simulink model "sampleModel2431_slicer"  (R2018a)
settings: Solver=FixedStepAuto  StartTime=0.0  StopTime=10.0  RelTol=1e-3
undefined symbols (not defined in the file): DiscIntNeverNeededParam, sigbuilder_block
libraries: simulink x433
(part 4 of 8)

== system sampleModel2431_slicer/cfblk240 ==
  cfblk1 : Inport
  cfblk13 : Inport  Port=2
  cfblk14 : Inport  Port=3
  Action Port : ActionPort  ActionType=else
  cfblk10 : DiscreteTransferFcn
  cfblk11 : UnitDelay  SampleTime=-1
  cfblk12 : If  SampleTime=1
  cfblk18 : Subsystem  TreatAsAtomicUnit=on
  cfblk19 : Subsystem  TreatAsAtomicUnit=on
  cfblk20 : Delay
  cfblk21 : Delay
  cfblk3 : simulink/Continuous/PID Controller (2DOF)  Controller=PID  TimeDomain=Discrete-time  SampleTime=-1  IntegratorMethod=Forward Euler  FilterMethod=Forward Euler  Form=Parallel  UseFilter=on  ControllerParametersSource=internal  P=1  I=1  D=0  N=100  b=1  c=1  InitialConditionSource=internal  InitialConditionForIntegrator=0  InitialConditionForFilter=0  ExternalReset=none  LimitOutput=off  UpperSaturationLimit=inf  LowerSaturationLimit=-inf  LinearizeAsGain=off  AntiWindupMode=none  Kb=1  TrackingMode=off  Kt=1  PParamMin=[]  PParamMax=[]  IParamMin=[]  IParamMax=[]  DParamMin=[]  DParamMax=[]  NParamMin=[]  NParamMax=[]  bParamMin=[]  bParamMax=[]  cParamMin=[]  cParamMax=[]  KbParamMin=[]  KbParamMax=[]  KtParamMin=[]  KtParamMax=[]  POutMin=[]  POutMax=[]  IOutMin=[]  IOutMax=[]  DOutMin=[]  DOutMax=[]  NOutMin=[]  NOutMax=[]  bOutMin=[]  bOutMax=[]  cOutMin=[]  cOutMax=[]  KbOutMin=[]  KbOutMax=[]  KtOutMin=[]  KtOutMax=[]  IntegratorOutMin=[]  IntegratorOutMax=[]  FilterOutMin=[]  FilterOutMax=[]  SumOutMin=[]  SumOutMax=[]  Sum1OutMin=[]  Sum1OutMax=[]  Sum2OutMin=[]  Sum2OutMax=[]  Sum3OutMin=[]  Sum3OutMax=[]  SumI1OutMin=[]  SumI1OutMax=[]  SumI2OutMin=[]  SumI2OutMax=[]  SumI3OutMin=[]  SumI3OutMax=[]  SumDOutMin=[]  SumDOutMax=[]  SaturationOutMin=[]  SaturationOutMax=[]  IntegratorContinuousStateAttributes=''  IntegratorStateMustResolveToSignalObject=off  IntegratorRTWStateStorageClass=Auto  FilterContinuousStateAttributes=''  FilterStateMustResolveToSignalObject=off  FilterRTWStateStorageClass=Auto  DifferentiatorICPrevScaledInput=0  DifferentiatorOutMin=[]  DifferentiatorOutMax=[]  FilterDiffOutCoefMin=[]  FilterDiffOutCoefMax=[]  SumDenOutMin=[]  SumDenOutMax=[]  SumNumOutMin=[]  SumNumOutMax=[]  ReciprocalOutMin=[]  ReciprocalOutMax=[]  DivideOutMin=[]  DivideOutMax=[]  TunerSelectOption=Transfer Function Based (PID Tuner App)
  cfblk4 : simulink/Discrete/Transfer Fcn First Order  PoleZ=0.95  ICPrevOutput=0.0  DoSatur=off
      settings: SourceProductName=Simulink
  cfblk5 : DiscreteFilter
  cfblk6 : Delay  ShowEnablePort=on
      settings: InputPortMap=u0,e6
  cfblk7 : simulink/Continuous/PID Controller (2DOF)  Controller=PID  TimeDomain=Discrete-time  SampleTime=-1  IntegratorMethod=Forward Euler  FilterMethod=Forward Euler  Form=Parallel  UseFilter=on  ControllerParametersSource=internal  P=1  I=1  D=0  N=100  b=1  c=1  InitialConditionSource=internal  InitialConditionForIntegrator=0  InitialConditionForFilter=0  ExternalReset=none  LimitOutput=off  UpperSaturationLimit=inf  LowerSaturationLimit=-inf  LinearizeAsGain=off  AntiWindupMode=none  Kb=1  TrackingMode=off  Kt=1  PParamMin=[]  PParamMax=[]  IParamMin=[]  IParamMax=[]  DParamMin=[]  DParamMax=[]  NParamMin=[]  NParamMax=[]  bParamMin=[]  bParamMax=[]  cParamMin=[]  cParamMax=[]  KbParamMin=[]  KbParamMax=[]  KtParamMin=[]  KtParamMax=[]  POutMin=[]  POutMax=[]  IOutMin=[]  IOutMax=[]  DOutMin=[]  DOutMax=[]  NOutMin=[]  NOutMax=[]  bOutMin=[]  bOutMax=[]  cOutMin=[]  cOutMax=[]  KbOutMin=[]  KbOutMax=[]  KtOutMin=[]  KtOutMax=[]  IntegratorOutMin=[]  IntegratorOutMax=[]  FilterOutMin=[]  FilterOutMax=[]  SumOutMin=[]  SumOutMax=[]  Sum1OutMin=[]  Sum1OutMax=[]  Sum2OutMin=[]  Sum2OutMax=[]  Sum3OutMin=[]  Sum3OutMax=[]  SumI1OutMin=[]  SumI1OutMax=[]  SumI2OutMin=[]  SumI2OutMax=[]  SumI3OutMin=[]  SumI3OutMax=[]  SumDOutMin=[]  SumDOutMax=[]  SaturationOutMin=[]  SaturationOutMax=[]  IntegratorContinuousStateAttributes=''  IntegratorStateMustResolveToSignalObject=off  IntegratorRTWStateStorageClass=Auto  FilterContinuousStateAttributes=''  FilterStateMustResolveToSignalObject=off  FilterRTWStateStorageClass=Auto  DifferentiatorICPrevScaledInput=0  DifferentiatorOutMin=[]  DifferentiatorOutMax=[]  FilterDiffOutCoefMin=[]  FilterDiffOutCoefMax=[]  SumDenOutMin=[]  SumDenOutMax=[]  SumNumOutMin=[]  SumNumOutMax=[]  ReciprocalOutMin=[]  ReciprocalOutMax=[]  DivideOutMin=[]  DivideOutMax=[]  TunerSelectOption=Transfer Function Based (PID Tuner App)
  cfblk8 : DiscreteStateSpace  SampleTime=-1
  cfblk9 : DiscreteTransferFcn
  cfblk2 : Outport
  cfblk15 : Outport  Port=2
  cfblk16 : Outport  Port=3
  cfblk17 : Outport  Port=4
  wires:
  cfblk18/1(cfblk2) -> cfblk15/1
  cfblk7/1 -> cfblk11/1
  cfblk4/1 -> cfblk9/1
  cfblk6/1 -> cfblk10/1
  cfblk5/1 -> cfblk17/1, cfblk2/1
  cfblk14/1 -> cfblk19/1(cfblk1)
  cfblk9/1 -> cfblk16/1
  cfblk11/1 -> cfblk5/1
  cfblk3/1 -> cfblk4/1
  cfblk8/1 -> cfblk6/1
  cfblk18/3(cfblk17) -> cfblk8/1
  cfblk13/1 -> cfblk18/1(cfblk1), cfblk3/2
  cfblk19/1(cfblk2) -> cfblk7/1
  cfblk19/2(cfblk7) -> cfblk7/2, cfblk18/2(cfblk15)
  cfblk1/1 -> cfblk3/1
  cfblk12/1 -> cfblk18/Action
  cfblk12/2 -> cfblk19/Action
  cfblk10/1 -> cfblk20/1
  cfblk20/1 -> cfblk6/2
  cfblk18/2(cfblk16) -> cfblk21/1
  cfblk21/1 -> cfblk12/1

== system sampleModel2431_slicer/cfblk241 ==
  cfblk1 : Inport
  cfblk9 : Inport  Port=2
  Action Port : ActionPort  ActionType=then
  cfblk11 : Delay
  cfblk3 : Delay  ShowEnablePort=on
      settings: InputPortMap=u0,e6
  cfblk4 : Delay  DelayLengthSource=Input port
      settings: InputPortMap=u0,p1
  cfblk5 : Delay  ShowEnablePort=on
      settings: InputPortMap=u0,e6
  cfblk6 : DiscreteFir
  cfblk7 : simulink/Discrete/Transfer Fcn First Order  PoleZ=0.95  ICPrevOutput=0.0  DoSatur=off
      settings: SourceProductName=Simulink
  cfblk8 : simulink/Discrete/Difference  ICPrevInput=0.0  OutMin=[]  OutMax=[]  OutDataTypeStr=Inherit: Inherit via back propagation  OutDataType=fixdt(1, 16)  OutScaling=2^-10  DoSatur=off
  cfblk2 : Outport
  cfblk10 : Outport  Port=2
  wires:
  cfblk5/1 -> cfblk6/1, cfblk8/1, cfblk10/1
  cfblk3/1 -> cfblk4/1
  cfblk9/1 -> cfblk7/1, cfblk3/2
  cfblk8/1 -> cfblk3/1
  cfblk1/1 -> cfblk4/2
  cfblk4/1 -> cfblk2/1
  cfblk7/1 -> cfblk5/2
  cfblk6/1 -> cfblk11/1
  cfblk11/1 -> cfblk5/1

== system sampleModel2431_slicer/cfblk242 ==
  cfblk1 : Inport
  Action Port : ActionPort  ActionType=else
  cfblk3 : simulink/Continuous/PID Controller  Controller=PID  TimeDomain=Discrete-time  SampleTime=-1  IntegratorMethod=Forward Euler  FilterMethod=Forward Euler  Form=Parallel  UseFilter=on  ControllerParametersSource=internal  P=1  I=1  D=0  N=100  InitialConditionSource=internal  InitialConditionForIntegrator=0  InitialConditionForFilter=0  ExternalReset=none  LimitOutput=off  UpperSaturationLimit=inf  LowerSaturationLimit=-inf  LinearizeAsGain=off  AntiWindupMode=none  Kb=1  TrackingMode=off  Kt=1  PParamMin=[]  PParamMax=[]  IParamMin=[]  IParamMax=[]  DParamMin=[]  DParamMax=[]  NParamMin=[]  NParamMax=[]  KbParamMin=[]  KbParamMax=[]  KtParamMin=[]  KtParamMax=[]  POutMin=[]  POutMax=[]  IOutMin=[]  IOutMax=[]  DOutMin=[]  DOutMax=[]  NOutMin=[]  NOutMax=[]  KbOutMin=[]  KbOutMax=[]  KtOutMin=[]  KtOutMax=[]  IntegratorOutMin=[]  IntegratorOutMax=[]  FilterOutMin=[]  FilterOutMax=[]  SumOutMin=[]  SumOutMax=[]  SumI1OutMin=[]  SumI1OutMax=[]  SumI2OutMin=[]  SumI2OutMax=[]  SumI3OutMin=[]  SumI3OutMax=[]  SumDOutMin=[]  SumDOutMax=[]  SaturationOutMin=[]  SaturationOutMax=[]  IntegratorContinuousStateAttributes=''  IntegratorStateMustResolveToSignalObject=off  IntegratorRTWStateStorageClass=Auto  FilterContinuousStateAttributes=''  FilterStateMustResolveToSignalObject=off  FilterRTWStateStorageClass=Auto  DifferentiatorICPrevScaledInput=0  DifferentiatorOutMin=[]  DifferentiatorOutMax=[]  FilterDiffOutCoefMin=[]  FilterDiffOutCoefMax=[]  SumDenOutMin=[]  SumDenOutMax=[]  SumNumOutMin=[]  SumNumOutMax=[]  ReciprocalOutMin=[]  ReciprocalOutMax=[]  DivideOutMin=[]  DivideOutMax=[]  TunerSelectOption=Transfer Function Based (PID Tuner App)
  cfblk4 : simulink/Discrete/Difference  ICPrevInput=0.0  OutMin=[]  OutMax=[]  OutDataTypeStr=Inherit: Inherit via back propagation  OutDataType=fixdt(1, 16)  OutScaling=2^-10  DoSatur=off
  cfblk5 : DiscreteStateSpace  SampleTime=-1
  cfblk6 : UnitDelay  SampleTime=-1
  cfblk7 : simulink/Discrete/Transfer Fcn Real Zero  ZeroZ=0.75  ICPrevInput=0.0  DoSatur=off
      settings: SourceProductName=Simulink  SourceProductBaseCode=SL
  cfblk8 : Delay
  cfblk9 : Delay
  cfblk2 : Outport
  cfblk10 : Outport  Port=2
  wires:
  cfblk3/1 -> cfblk2/1
  cfblk6/1 -> cfblk7/1
  cfblk4/1 -> cfblk8/1
  cfblk7/1 -> cfblk9/1
  cfblk5/1 -> cfblk4/1
  cfblk1/1 -> cfblk6/1
  cfblk8/1 -> cfblk10/1, cfblk3/1
  cfblk9/1 -> cfblk5/1

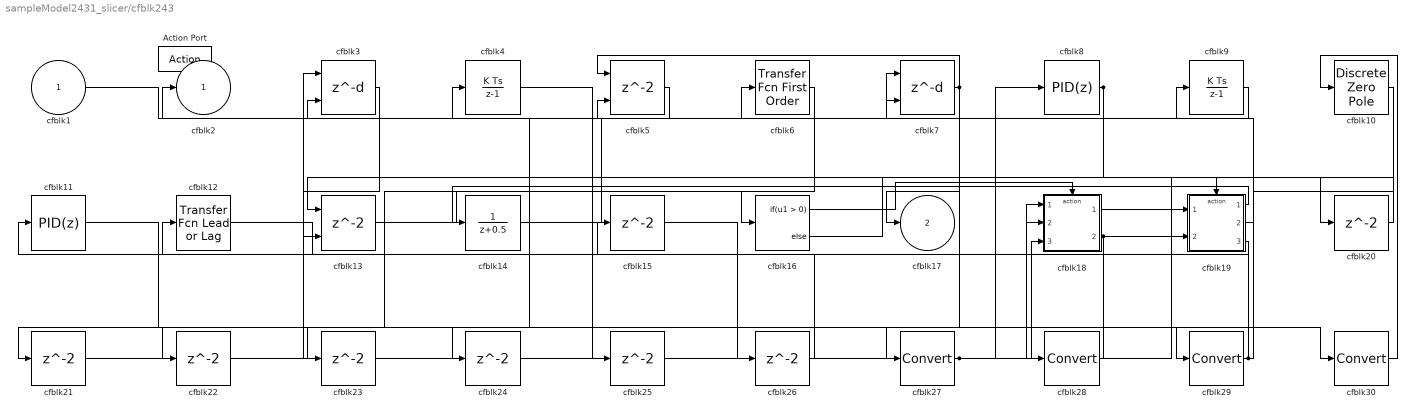
== system sampleModel2431_slicer/cfblk243 ==
  cfblk1 : Inport
  Action Port : ActionPort  ActionType=then
  cfblk10 : DiscreteZeroPole  Poles=[0 0.5]  Gain=1  SampleTime=-1
  cfblk11 : simulink/Continuous/PID Controller  Controller=PID  TimeDomain=Discrete-time  SampleTime=-1  IntegratorMethod=Forward Euler  FilterMethod=Forward Euler  Form=Parallel  UseFilter=on  ControllerParametersSource=internal  P=1  I=1  D=0  N=100  InitialConditionSource=internal  InitialConditionForIntegrator=0  InitialConditionForFilter=0  ExternalReset=none  LimitOutput=off  UpperSaturationLimit=inf  LowerSaturationLimit=-inf  LinearizeAsGain=off  AntiWindupMode=none  Kb=1  TrackingMode=off  Kt=1  PParamMin=[]  PParamMax=[]  IParamMin=[]  IParamMax=[]  DParamMin=[]  DParamMax=[]  NParamMin=[]  NParamMax=[]  KbParamMin=[]  KbParamMax=[]  KtParamMin=[]  KtParamMax=[]  POutMin=[]  POutMax=[]  IOutMin=[]  IOutMax=[]  DOutMin=[]  DOutMax=[]  NOutMin=[]  NOutMax=[]  KbOutMin=[]  KbOutMax=[]  KtOutMin=[]  KtOutMax=[]  IntegratorOutMin=[]  IntegratorOutMax=[]  FilterOutMin=[]  FilterOutMax=[]  SumOutMin=[]  SumOutMax=[]  SumI1OutMin=[]  SumI1OutMax=[]  SumI2OutMin=[]  SumI2OutMax=[]  SumI3OutMin=[]  SumI3OutMax=[]  SumDOutMin=[]  SumDOutMax=[]  SaturationOutMin=[]  SaturationOutMax=[]  IntegratorContinuousStateAttributes=''  IntegratorStateMustResolveToSignalObject=off  IntegratorRTWStateStorageClass=Auto  FilterContinuousStateAttributes=''  FilterStateMustResolveToSignalObject=off  FilterRTWStateStorageClass=Auto  DifferentiatorICPrevScaledInput=0  DifferentiatorOutMin=[]  DifferentiatorOutMax=[]  FilterDiffOutCoefMin=[]  FilterDiffOutCoefMax=[]  SumDenOutMin=[]  SumDenOutMax=[]  SumNumOutMin=[]  SumNumOutMax=[]  ReciprocalOutMin=[]  ReciprocalOutMax=[]  DivideOutMin=[]  DivideOutMax=[]  TunerSelectOption=Transfer Function Based (PID Tuner App)
  cfblk12 : simulink/Discrete/Transfer Fcn Lead or Lag  PoleZ=0.95  ZeroZ=0.75  ICPrevOutput=0.0  ICPrevInput=0.0  DoSatur=off
      settings: SourceProductName=Simulink  SourceProductBaseCode=SL
  cfblk13 : Delay  ShowEnablePort=on
      settings: InputPortMap=u0,e6
  cfblk14 : DiscreteTransferFcn
  cfblk{15,20..26} (8 alike) : Delay
  cfblk16 : If  SampleTime=1
  cfblk18 : Subsystem  TreatAsAtomicUnit=on
  cfblk19 : Subsystem  TreatAsAtomicUnit=on
  cfblk{27..30} (4 alike) : DataTypeConversion
  cfblk3 : Delay  DelayLengthSource=Input port
      settings: InputPortMap=u0,p1
  cfblk4 : DiscreteIntegrator  SampleTime=-1  ICPrevOutput=DiscIntNeverNeededParam  ICPrevScaledInput=DiscIntNeverNeededParam
  cfblk5 : Delay  ShowEnablePort=on
      settings: InputPortMap=u0,e6
  cfblk6 : simulink/Discrete/Transfer Fcn First Order  PoleZ=0.95  ICPrevOutput=0.0  DoSatur=off
      settings: SourceProductName=Simulink
  cfblk7 : Delay  DelayLengthSource=Input port
      settings: InputPortMap=u0,p1
  cfblk8 : simulink/Continuous/PID Controller  Controller=PID  TimeDomain=Discrete-time  SampleTime=-1  IntegratorMethod=Forward Euler  FilterMethod=Forward Euler  Form=Parallel  UseFilter=on  ControllerParametersSource=internal  P=1  I=1  D=0  N=100  InitialConditionSource=internal  InitialConditionForIntegrator=0  InitialConditionForFilter=0  ExternalReset=none  LimitOutput=off  UpperSaturationLimit=inf  LowerSaturationLimit=-inf  LinearizeAsGain=off  AntiWindupMode=none  Kb=1  TrackingMode=off  Kt=1  PParamMin=[]  PParamMax=[]  IParamMin=[]  IParamMax=[]  DParamMin=[]  DParamMax=[]  NParamMin=[]  NParamMax=[]  KbParamMin=[]  KbParamMax=[]  KtParamMin=[]  KtParamMax=[]  POutMin=[]  POutMax=[]  IOutMin=[]  IOutMax=[]  DOutMin=[]  DOutMax=[]  NOutMin=[]  NOutMax=[]  KbOutMin=[]  KbOutMax=[]  KtOutMin=[]  KtOutMax=[]  IntegratorOutMin=[]  IntegratorOutMax=[]  FilterOutMin=[]  FilterOutMax=[]  SumOutMin=[]  SumOutMax=[]  SumI1OutMin=[]  SumI1OutMax=[]  SumI2OutMin=[]  SumI2OutMax=[]  SumI3OutMin=[]  SumI3OutMax=[]  SumDOutMin=[]  SumDOutMax=[]  SaturationOutMin=[]  SaturationOutMax=[]  IntegratorContinuousStateAttributes=''  IntegratorStateMustResolveToSignalObject=off  IntegratorRTWStateStorageClass=Auto  FilterContinuousStateAttributes=''  FilterStateMustResolveToSignalObject=off  FilterRTWStateStorageClass=Auto  DifferentiatorICPrevScaledInput=0  DifferentiatorOutMin=[]  DifferentiatorOutMax=[]  FilterDiffOutCoefMin=[]  FilterDiffOutCoefMax=[]  SumDenOutMin=[]  SumDenOutMax=[]  SumNumOutMin=[]  SumNumOutMax=[]  ReciprocalOutMin=[]  ReciprocalOutMax=[]  DivideOutMin=[]  DivideOutMax=[]  TunerSelectOption=Transfer Function Based (PID Tuner App)
  cfblk9 : DiscreteIntegrator  SampleTime=-1  ICPrevOutput=DiscIntNeverNeededParam  ICPrevScaledInput=DiscIntNeverNeededParam
  cfblk2 : Outport
  cfblk17 : Outport  Port=2
  wires:
  cfblk14/1 -> cfblk7/1
  cfblk12/1 -> cfblk15/1
  cfblk9/1 -> cfblk7/2
  cfblk7/1 -> cfblk5/1, cfblk17/1, cfblk22/1
  cfblk5/1 -> cfblk2/1
  cfblk18/2(cfblk16) -> cfblk19/2(cfblk11), cfblk21/1
  cfblk10/1 -> cfblk29/1
  cfblk11/1 -> cfblk27/1
  cfblk13/1 -> cfblk16/1
  cfblk8/1 -> cfblk5/2, cfblk24/1
  cfblk1/1 -> cfblk3/2
  cfblk3/1 -> cfblk13/2
  cfblk19/1(cfblk2) -> cfblk14/1
  cfblk19/2(cfblk12) -> cfblk6/1
  cfblk16/1 -> cfblk18/Action
  cfblk16/2 -> cfblk19/Action
  cfblk18/1(cfblk2) -> cfblk20/1
  cfblk20/1 -> cfblk13/1
  cfblk21/1 -> cfblk3/1
  cfblk22/1 -> cfblk18/3(cfblk15)
  cfblk6/1 -> cfblk23/1
  cfblk23/1 -> cfblk18/1(cfblk1)
  cfblk24/1 -> cfblk18/2(cfblk14)
  cfblk4/1 -> cfblk25/1
  cfblk25/1 -> cfblk19/1(cfblk1)
  cfblk15/1 -> cfblk26/1
  cfblk26/1 -> cfblk12/1
  cfblk27/1 -> cfblk8/1, cfblk30/1
  cfblk19/3(cfblk13) -> cfblk28/1
  cfblk28/1 -> cfblk11/1
  cfblk29/1 -> cfblk4/1, cfblk9/1
  cfblk30/1 -> cfblk10/1

== system sampleModel2431_slicer/cfblk244 ==
  cfblk1 : Inport
  Action Port : ActionPort  ActionType=else
  cfblk10 : Delay
  cfblk11 : Delay
  cfblk12 : Delay
  cfblk3 : UnitDelay  SampleTime=-1
  cfblk4 : simulink/Discrete/Transfer Fcn Real Zero  ZeroZ=0.75  ICPrevInput=0.0  DoSatur=off
      settings: SourceProductName=Simulink  SourceProductBaseCode=SL
  cfblk5 : simulink/Discrete/Transfer Fcn Lead or Lag  PoleZ=0.95  ZeroZ=0.75  ICPrevOutput=0.0  ICPrevInput=0.0  DoSatur=off
      settings: SourceProductName=Simulink  SourceProductBaseCode=SL
  cfblk6 : DiscreteFir
  cfblk7 : If  SampleTime=1
  cfblk8 : Subsystem  TreatAsAtomicUnit=on
  cfblk9 : Subsystem  TreatAsAtomicUnit=on
  cfblk2 : Outport
  wires:
  cfblk1/1 -> cfblk5/1
  cfblk4/1 -> cfblk3/1, cfblk11/1
  cfblk5/1 -> cfblk2/1, cfblk6/1
  cfblk6/1 -> cfblk8/2(cfblk13)
  cfblk8/1(cfblk2) -> cfblk4/1
  cfblk8/2(cfblk15) -> cfblk9/1(cfblk1)
  cfblk8/3(cfblk16) -> cfblk9/2(cfblk10)
  cfblk7/1 -> cfblk8/Action
  cfblk7/2 -> cfblk9/Action
  cfblk3/1 -> cfblk10/1
  cfblk10/1 -> cfblk8/1(cfblk1)
  cfblk11/1 -> cfblk8/3(cfblk14)
  cfblk9/1(cfblk2) -> cfblk12/1
  cfblk12/1 -> cfblk7/1

== system sampleModel2431_slicer/cfblk245 ==
  cfblk1 : Inport
  cfblk12 : Inport  Port=2
  cfblk13 : Inport  Port=3
  Action Port : ActionPort  ActionType=then
  cfblk10 : If  SampleTime=1
  cfblk11 : If  SampleTime=1
  cfblk14 : Subsystem  TreatAsAtomicUnit=on
  cfblk15 : Subsystem  TreatAsAtomicUnit=on
  cfblk16 : Subsystem  TreatAsAtomicUnit=on
  cfblk17 : Subsystem  TreatAsAtomicUnit=on
  cfblk{18..21} (4 alike) : Delay
  cfblk3 : DiscreteIntegrator  SampleTime=-1  ICPrevOutput=DiscIntNeverNeededParam  ICPrevScaledInput=DiscIntNeverNeededParam
  cfblk4 : simulink/Discrete/Transfer Fcn First Order  PoleZ=0.95  ICPrevOutput=0.0  DoSatur=off
      settings: SourceProductName=Simulink
  cfblk5 : simulink/Discrete/Difference  ICPrevInput=0.0  OutMin=[]  OutMax=[]  OutDataTypeStr=Inherit: Inherit via back propagation  OutDataType=fixdt(1, 16)  OutScaling=2^-10  DoSatur=off
  cfblk6 : DiscreteStateSpace  SampleTime=-1
  cfblk7 : simulink/Discrete/Tapped Delay  vinit=0.0  samptime=-1  NumDelays=1  DelayOrder=Oldest  includeCurrent=off
  cfblk8 : Delay  ShowEnablePort=on
      settings: InputPortMap=u0,e6
  cfblk9 : Delay  ShowEnablePort=on
      settings: InputPortMap=u0,e6
  cfblk2 : Outport
  wires:
  cfblk9/1 -> cfblk6/1
  cfblk7/1 -> cfblk15/1(cfblk1), cfblk8/2, cfblk15/4(cfblk11), cfblk20/1
  cfblk1/1 -> cfblk16/1(cfblk1), cfblk17/3(cfblk16)
  cfblk16/1(cfblk2) -> cfblk10/1
  cfblk12/1 -> cfblk16/2(cfblk8)
  cfblk15/1(cfblk2) -> cfblk5/1
  cfblk3/1 -> cfblk8/1
  cfblk8/1 -> cfblk9/1
  cfblk15/2(cfblk12) -> cfblk3/1
  cfblk4/1 -> cfblk14/1(cfblk1), cfblk7/1
  cfblk13/1 -> cfblk9/2
  cfblk16/2(cfblk9) -> cfblk4/1, cfblk14/2(cfblk11), cfblk21/1
  cfblk14/1(cfblk2) -> cfblk15/3(cfblk10)
  cfblk17/1(cfblk2) -> cfblk2/1
  cfblk10/1 -> cfblk14/Action
  cfblk10/2 -> cfblk15/Action
  cfblk11/1 -> cfblk16/Action
  cfblk11/2 -> cfblk17/Action
  cfblk5/1 -> cfblk18/1
  cfblk18/1 -> cfblk17/1(cfblk1)
  cfblk6/1 -> cfblk19/1
  cfblk19/1 -> cfblk15/2(cfblk9)
  cfblk20/1 -> cfblk17/2(cfblk15)
  cfblk21/1 -> cfblk11/1

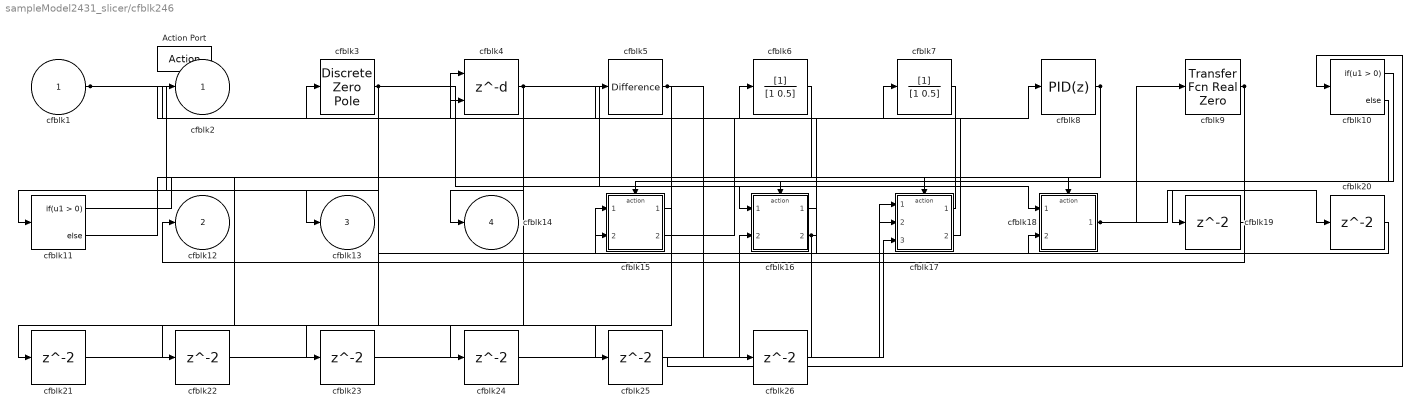
== system sampleModel2431_slicer/cfblk246 ==
  cfblk1 : Inport
  Action Port : ActionPort  ActionType=else
  cfblk10 : If  SampleTime=1
  cfblk11 : If  SampleTime=1
  cfblk15 : Subsystem  TreatAsAtomicUnit=on
  cfblk16 : Subsystem  TreatAsAtomicUnit=on
  cfblk17 : Subsystem  TreatAsAtomicUnit=on
  cfblk18 : Subsystem  TreatAsAtomicUnit=on
  cfblk{19..26} (8 alike) : Delay
  cfblk3 : DiscreteZeroPole  Poles=[0 0.5]  Gain=1  SampleTime=-1
  cfblk4 : Delay  DelayLengthSource=Input port
      settings: InputPortMap=u0,p1
  cfblk5 : simulink/Discrete/Difference  ICPrevInput=0.0  OutMin=[]  OutMax=[]  OutDataTypeStr=Inherit: Inherit via back propagation  OutDataType=fixdt(1, 16)  OutScaling=2^-10  DoSatur=off
  cfblk6 : DiscreteFilter
  cfblk7 : DiscreteFilter
  cfblk8 : simulink/Continuous/PID Controller  Controller=PID  TimeDomain=Discrete-time  SampleTime=-1  IntegratorMethod=Forward Euler  FilterMethod=Forward Euler  Form=Parallel  UseFilter=on  ControllerParametersSource=internal  P=1  I=1  D=0  N=100  InitialConditionSource=internal  InitialConditionForIntegrator=0  InitialConditionForFilter=0  ExternalReset=none  LimitOutput=off  UpperSaturationLimit=inf  LowerSaturationLimit=-inf  LinearizeAsGain=off  AntiWindupMode=none  Kb=1  TrackingMode=off  Kt=1  PParamMin=[]  PParamMax=[]  IParamMin=[]  IParamMax=[]  DParamMin=[]  DParamMax=[]  NParamMin=[]  NParamMax=[]  KbParamMin=[]  KbParamMax=[]  KtParamMin=[]  KtParamMax=[]  POutMin=[]  POutMax=[]  IOutMin=[]  IOutMax=[]  DOutMin=[]  DOutMax=[]  NOutMin=[]  NOutMax=[]  KbOutMin=[]  KbOutMax=[]  KtOutMin=[]  KtOutMax=[]  IntegratorOutMin=[]  IntegratorOutMax=[]  FilterOutMin=[]  FilterOutMax=[]  SumOutMin=[]  SumOutMax=[]  SumI1OutMin=[]  SumI1OutMax=[]  SumI2OutMin=[]  SumI2OutMax=[]  SumI3OutMin=[]  SumI3OutMax=[]  SumDOutMin=[]  SumDOutMax=[]  SaturationOutMin=[]  SaturationOutMax=[]  IntegratorContinuousStateAttributes=''  IntegratorStateMustResolveToSignalObject=off  IntegratorRTWStateStorageClass=Auto  FilterContinuousStateAttributes=''  FilterStateMustResolveToSignalObject=off  FilterRTWStateStorageClass=Auto  DifferentiatorICPrevScaledInput=0  DifferentiatorOutMin=[]  DifferentiatorOutMax=[]  FilterDiffOutCoefMin=[]  FilterDiffOutCoefMax=[]  SumDenOutMin=[]  SumDenOutMax=[]  SumNumOutMin=[]  SumNumOutMax=[]  ReciprocalOutMin=[]  ReciprocalOutMax=[]  DivideOutMin=[]  DivideOutMax=[]  TunerSelectOption=Transfer Function Based (PID Tuner App)
  cfblk9 : simulink/Discrete/Transfer Fcn Real Zero  ZeroZ=0.75  ICPrevInput=0.0  DoSatur=off
      settings: SourceProductName=Simulink  SourceProductBaseCode=SL
  cfblk2 : Outport
  cfblk12 : Outport  Port=2
  cfblk13 : Outport  Port=3
  cfblk14 : Outport  Port=4
  wires:
  cfblk1/1 -> cfblk13/1, cfblk4/1
  cfblk4/1 -> cfblk16/1(cfblk1), cfblk14/1
  cfblk16/1(cfblk2) -> cfblk3/1
  cfblk8/1 -> cfblk23/1, cfblk24/1
  cfblk15/2(cfblk12) -> cfblk8/1
  cfblk5/1 -> cfblk25/1, cfblk26/1
  cfblk16/2(cfblk17) -> cfblk5/1, cfblk15/1(cfblk1)
  cfblk7/1 -> cfblk2/1
  cfblk18/1(cfblk2) -> cfblk9/1, cfblk20/1
  cfblk9/1 -> cfblk12/1, cfblk19/1
  cfblk17/1(cfblk2) -> cfblk6/1
  cfblk3/1 -> cfblk18/1(cfblk1), cfblk11/1
  cfblk17/2(cfblk9) -> cfblk7/1
  cfblk10/1 -> cfblk15/Action
  cfblk10/2 -> cfblk16/Action
  cfblk11/1 -> cfblk17/Action
  cfblk11/2 -> cfblk18/Action
  cfblk19/1 -> cfblk18/2(cfblk10)
  cfblk20/1 -> cfblk15/2(cfblk11)
  cfblk15/1(cfblk2) -> cfblk21/1
  cfblk21/1 -> cfblk17/1(cfblk1)
  cfblk6/1 -> cfblk22/1
  cfblk22/1 -> cfblk17/2(cfblk7)
  cfblk23/1 -> cfblk17/3(cfblk8)
  cfblk24/1 -> cfblk16/2(cfblk16)
  cfblk25/1 -> cfblk10/1
  cfblk26/1 -> cfblk4/2

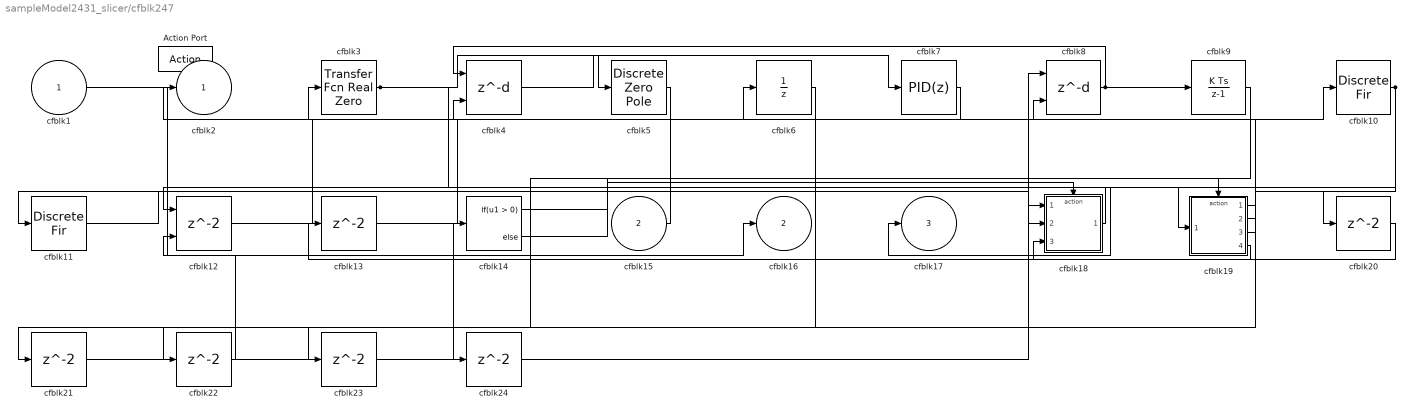
== system sampleModel2431_slicer/cfblk247 ==
  cfblk1 : Inport
  cfblk15 : Inport  Port=2
  Action Port : ActionPort  ActionType=then
  cfblk10 : DiscreteFir
  cfblk11 : DiscreteFir
  cfblk12 : Delay  ShowEnablePort=on
      settings: InputPortMap=u0,e6
  cfblk{13,20..24} (6 alike) : Delay
  cfblk14 : If  SampleTime=1
  cfblk18 : Subsystem  TreatAsAtomicUnit=on
  cfblk19 : Subsystem  TreatAsAtomicUnit=on
  cfblk3 : simulink/Discrete/Transfer Fcn Real Zero  ZeroZ=0.75  ICPrevInput=0.0  DoSatur=off
      settings: SourceProductName=Simulink  SourceProductBaseCode=SL
  cfblk4 : Delay  DelayLengthSource=Input port
      settings: InputPortMap=u0,p1
  cfblk5 : DiscreteZeroPole  Poles=[0 0.5]  Gain=1  SampleTime=-1
  cfblk6 : UnitDelay  SampleTime=-1
  cfblk7 : simulink/Continuous/PID Controller  Controller=PID  TimeDomain=Discrete-time  SampleTime=-1  IntegratorMethod=Forward Euler  FilterMethod=Forward Euler  Form=Parallel  UseFilter=on  ControllerParametersSource=internal  P=1  I=1  D=0  N=100  InitialConditionSource=internal  InitialConditionForIntegrator=0  InitialConditionForFilter=0  ExternalReset=none  LimitOutput=off  UpperSaturationLimit=inf  LowerSaturationLimit=-inf  LinearizeAsGain=off  AntiWindupMode=none  Kb=1  TrackingMode=off  Kt=1  PParamMin=[]  PParamMax=[]  IParamMin=[]  IParamMax=[]  DParamMin=[]  DParamMax=[]  NParamMin=[]  NParamMax=[]  KbParamMin=[]  KbParamMax=[]  KtParamMin=[]  KtParamMax=[]  POutMin=[]  POutMax=[]  IOutMin=[]  IOutMax=[]  DOutMin=[]  DOutMax=[]  NOutMin=[]  NOutMax=[]  KbOutMin=[]  KbOutMax=[]  KtOutMin=[]  KtOutMax=[]  IntegratorOutMin=[]  IntegratorOutMax=[]  FilterOutMin=[]  FilterOutMax=[]  SumOutMin=[]  SumOutMax=[]  SumI1OutMin=[]  SumI1OutMax=[]  SumI2OutMin=[]  SumI2OutMax=[]  SumI3OutMin=[]  SumI3OutMax=[]  SumDOutMin=[]  SumDOutMax=[]  SaturationOutMin=[]  SaturationOutMax=[]  IntegratorContinuousStateAttributes=''  IntegratorStateMustResolveToSignalObject=off  IntegratorRTWStateStorageClass=Auto  FilterContinuousStateAttributes=''  FilterStateMustResolveToSignalObject=off  FilterRTWStateStorageClass=Auto  DifferentiatorICPrevScaledInput=0  DifferentiatorOutMin=[]  DifferentiatorOutMax=[]  FilterDiffOutCoefMin=[]  FilterDiffOutCoefMax=[]  SumDenOutMin=[]  SumDenOutMax=[]  SumNumOutMin=[]  SumNumOutMax=[]  ReciprocalOutMin=[]  ReciprocalOutMax=[]  DivideOutMin=[]  DivideOutMax=[]  TunerSelectOption=Transfer Function Based (PID Tuner App)
  cfblk8 : Delay  DelayLengthSource=Input port
      settings: InputPortMap=u0,p1
  cfblk9 : DiscreteIntegrator  SampleTime=-1  ICPrevOutput=DiscIntNeverNeededParam  ICPrevScaledInput=DiscIntNeverNeededParam
  cfblk2 : Outport
  cfblk16 : Outport  Port=2
  cfblk17 : Outport  Port=3
  wires:
  cfblk12/1 -> cfblk10/1
  cfblk15/1 -> cfblk3/1
  cfblk3/1 -> cfblk5/1, cfblk19/1(cfblk1)
  cfblk1/1 -> cfblk16/1
  cfblk8/1 -> cfblk4/1, cfblk9/1
  cfblk10/1 -> cfblk17/1, cfblk20/1, cfblk21/1
  cfblk18/1(cfblk2) -> cfblk12/1
  cfblk4/1 -> cfblk7/1
  cfblk5/1 -> cfblk11/1
  cfblk11/1 -> cfblk18/2(cfblk11)
  cfblk7/1 -> cfblk2/1
  cfblk19/2(cfblk5) -> cfblk4/2
  cfblk13/1 -> cfblk8/2
  cfblk19/3(cfblk6) -> cfblk6/1
  cfblk19/4(cfblk7) -> cfblk13/1
  cfblk14/1 -> cfblk18/Action
  cfblk14/2 -> cfblk19/Action
  cfblk20/1 -> cfblk18/3(cfblk12)
  cfblk21/1 -> cfblk14/1
  cfblk19/1(cfblk2) -> cfblk22/1
  cfblk22/1 -> cfblk12/2
  cfblk6/1 -> cfblk23/1
  cfblk23/1 -> cfblk18/1(cfblk1)
  cfblk9/1 -> cfblk24/1
  cfblk24/1 -> cfblk8/1

== system sampleModel2431_slicer/cfblk248 ==
  cfblk1 : Inport
  cfblk8 : Inport  Port=2
  Action Port : ActionPort  ActionType=else
  cfblk3 : Delay  ShowEnablePort=on
      settings: InputPortMap=u0,e6
  cfblk4 : Delay  DelayLengthSource=Input port
      settings: InputPortMap=u0,p1
  cfblk5 : Delay
  cfblk6 : DiscreteStateSpace  SampleTime=-1
  cfblk7 : simulink/Discrete/Transfer Fcn Lead or Lag  PoleZ=0.95  ZeroZ=0.75  ICPrevOutput=0.0  ICPrevInput=0.0  DoSatur=off
      settings: SourceProductName=Simulink  SourceProductBaseCode=SL
  cfblk2 : Outport
  cfblk9 : Outport  Port=2
  wires:
  cfblk7/1 -> cfblk4/1, cfblk4/2
  cfblk4/1 -> cfblk9/1
  cfblk8/1 -> cfblk6/1
  cfblk6/1 -> cfblk3/1, cfblk3/2
  cfblk1/1 -> cfblk2/1
  cfblk3/1 -> cfblk5/1
  cfblk5/1 -> cfblk7/1

== system sampleModel2431_slicer/cfblk249 ==
  cfblk1 : Inport
  cfblk12 : Inport  Port=2
  Action Port : ActionPort  ActionType=then
  cfblk10 : DiscreteFilter
  cfblk11 : DiscreteTransferFcn
  cfblk13 : Delay
  cfblk3 : Delay
  cfblk4 : simulink/Discrete/Difference  ICPrevInput=0.0  OutMin=[]  OutMax=[]  OutDataTypeStr=Inherit: Inherit via back propagation  OutDataType=fixdt(1, 16)  OutScaling=2^-10  DoSatur=off
  cfblk5 : simulink/Discrete/Transfer Fcn Lead or Lag  PoleZ=0.95  ZeroZ=0.75  ICPrevOutput=0.0  ICPrevInput=0.0  DoSatur=off
      settings: SourceProductName=Simulink  SourceProductBaseCode=SL
  cfblk6 : DiscreteFir
  cfblk7 : DiscreteIntegrator  SampleTime=-1  ICPrevOutput=DiscIntNeverNeededParam  ICPrevScaledInput=DiscIntNeverNeededParam
  cfblk8 : simulink/Continuous/PID Controller  Controller=PID  TimeDomain=Discrete-time  SampleTime=-1  IntegratorMethod=Forward Euler  FilterMethod=Forward Euler  Form=Parallel  UseFilter=on  ControllerParametersSource=internal  P=1  I=1  D=0  N=100  InitialConditionSource=internal  InitialConditionForIntegrator=0  InitialConditionForFilter=0  ExternalReset=none  LimitOutput=off  UpperSaturationLimit=inf  LowerSaturationLimit=-inf  LinearizeAsGain=off  AntiWindupMode=none  Kb=1  TrackingMode=off  Kt=1  PParamMin=[]  PParamMax=[]  IParamMin=[]  IParamMax=[]  DParamMin=[]  DParamMax=[]  NParamMin=[]  NParamMax=[]  KbParamMin=[]  KbParamMax=[]  KtParamMin=[]  KtParamMax=[]  POutMin=[]  POutMax=[]  IOutMin=[]  IOutMax=[]  DOutMin=[]  DOutMax=[]  NOutMin=[]  NOutMax=[]  KbOutMin=[]  KbOutMax=[]  KtOutMin=[]  KtOutMax=[]  IntegratorOutMin=[]  IntegratorOutMax=[]  FilterOutMin=[]  FilterOutMax=[]  SumOutMin=[]  SumOutMax=[]  SumI1OutMin=[]  SumI1OutMax=[]  SumI2OutMin=[]  SumI2OutMax=[]  SumI3OutMin=[]  SumI3OutMax=[]  SumDOutMin=[]  SumDOutMax=[]  SaturationOutMin=[]  SaturationOutMax=[]  IntegratorContinuousStateAttributes=''  IntegratorStateMustResolveToSignalObject=off  IntegratorRTWStateStorageClass=Auto  FilterContinuousStateAttributes=''  FilterStateMustResolveToSignalObject=off  FilterRTWStateStorageClass=Auto  DifferentiatorICPrevScaledInput=0  DifferentiatorOutMin=[]  DifferentiatorOutMax=[]  FilterDiffOutCoefMin=[]  FilterDiffOutCoefMax=[]  SumDenOutMin=[]  SumDenOutMax=[]  SumNumOutMin=[]  SumNumOutMax=[]  ReciprocalOutMin=[]  ReciprocalOutMax=[]  DivideOutMin=[]  DivideOutMax=[]  TunerSelectOption=Transfer Function Based (PID Tuner App)
  cfblk9 : DiscreteStateSpace  SampleTime=-1
  cfblk2 : Outport
  wires:
  cfblk1/1 -> cfblk7/1
  cfblk10/1 -> cfblk2/1
  cfblk11/1 -> cfblk6/1
  cfblk12/1 -> cfblk11/1
  cfblk7/1 -> cfblk4/1
  cfblk4/1 -> cfblk9/1
  cfblk5/1 -> cfblk8/1
  cfblk3/1 -> cfblk10/1
  cfblk6/1 -> cfblk3/1
  cfblk8/1 -> cfblk13/1
  cfblk13/1 -> cfblk5/1

== system sampleModel2431_slicer/cfblk250 ==
  cfblk1 : Inport
  cfblk12 : Inport  Port=2
  cfblk13 : Inport  Port=3
  cfblk14 : Inport  Port=4
  Action Port : ActionPort  ActionType=else
  cfblk10 : DiscreteTransferFcn
  cfblk11 : If  SampleTime=1
  cfblk16 : Subsystem  TreatAsAtomicUnit=on
  cfblk17 : Subsystem  TreatAsAtomicUnit=on
  cfblk18 : Delay
  cfblk3 : DiscreteIntegrator  SampleTime=-1  ICPrevOutput=DiscIntNeverNeededParam  ICPrevScaledInput=DiscIntNeverNeededParam
  cfblk4 : simulink/Continuous/PID Controller (2DOF)  Controller=PID  TimeDomain=Discrete-time  SampleTime=-1  IntegratorMethod=Forward Euler  FilterMethod=Forward Euler  Form=Parallel  UseFilter=on  ControllerParametersSource=internal  P=1  I=1  D=0  N=100  b=1  c=1  InitialConditionSource=internal  InitialConditionForIntegrator=0  InitialConditionForFilter=0  ExternalReset=none  LimitOutput=off  UpperSaturationLimit=inf  LowerSaturationLimit=-inf  LinearizeAsGain=off  AntiWindupMode=none  Kb=1  TrackingMode=off  Kt=1  PParamMin=[]  PParamMax=[]  IParamMin=[]  IParamMax=[]  DParamMin=[]  DParamMax=[]  NParamMin=[]  NParamMax=[]  bParamMin=[]  bParamMax=[]  cParamMin=[]  cParamMax=[]  KbParamMin=[]  KbParamMax=[]  KtParamMin=[]  KtParamMax=[]  POutMin=[]  POutMax=[]  IOutMin=[]  IOutMax=[]  DOutMin=[]  DOutMax=[]  NOutMin=[]  NOutMax=[]  bOutMin=[]  bOutMax=[]  cOutMin=[]  cOutMax=[]  KbOutMin=[]  KbOutMax=[]  KtOutMin=[]  KtOutMax=[]  IntegratorOutMin=[]  IntegratorOutMax=[]  FilterOutMin=[]  FilterOutMax=[]  SumOutMin=[]  SumOutMax=[]  Sum1OutMin=[]  Sum1OutMax=[]  Sum2OutMin=[]  Sum2OutMax=[]  Sum3OutMin=[]  Sum3OutMax=[]  SumI1OutMin=[]  SumI1OutMax=[]  SumI2OutMin=[]  SumI2OutMax=[]  SumI3OutMin=[]  SumI3OutMax=[]  SumDOutMin=[]  SumDOutMax=[]  SaturationOutMin=[]  SaturationOutMax=[]  IntegratorContinuousStateAttributes=''  IntegratorStateMustResolveToSignalObject=off  IntegratorRTWStateStorageClass=Auto  FilterContinuousStateAttributes=''  FilterStateMustResolveToSignalObject=off  FilterRTWStateStorageClass=Auto  DifferentiatorICPrevScaledInput=0  DifferentiatorOutMin=[]  DifferentiatorOutMax=[]  FilterDiffOutCoefMin=[]  FilterDiffOutCoefMax=[]  SumDenOutMin=[]  SumDenOutMax=[]  SumNumOutMin=[]  SumNumOutMax=[]  ReciprocalOutMin=[]  ReciprocalOutMax=[]  DivideOutMin=[]  DivideOutMax=[]  TunerSelectOption=Transfer Function Based (PID Tuner App)
  cfblk5 : DiscreteIntegrator  SampleTime=-1  ICPrevOutput=DiscIntNeverNeededParam  ICPrevScaledInput=DiscIntNeverNeededParam
  cfblk6 : simulink/Discrete/Transfer Fcn First Order  PoleZ=0.95  ICPrevOutput=0.0  DoSatur=off
      settings: SourceProductName=Simulink
  cfblk7 : simulink/Continuous/PID Controller (2DOF)  Controller=PID  TimeDomain=Discrete-time  SampleTime=-1  IntegratorMethod=Forward Euler  FilterMethod=Forward Euler  Form=Parallel  UseFilter=on  ControllerParametersSource=internal  P=1  I=1  D=0  N=100  b=1  c=1  InitialConditionSource=internal  InitialConditionForIntegrator=0  InitialConditionForFilter=0  ExternalReset=none  LimitOutput=off  UpperSaturationLimit=inf  LowerSaturationLimit=-inf  LinearizeAsGain=off  AntiWindupMode=none  Kb=1  TrackingMode=off  Kt=1  PParamMin=[]  PParamMax=[]  IParamMin=[]  IParamMax=[]  DParamMin=[]  DParamMax=[]  NParamMin=[]  NParamMax=[]  bParamMin=[]  bParamMax=[]  cParamMin=[]  cParamMax=[]  KbParamMin=[]  KbParamMax=[]  KtParamMin=[]  KtParamMax=[]  POutMin=[]  POutMax=[]  IOutMin=[]  IOutMax=[]  DOutMin=[]  DOutMax=[]  NOutMin=[]  NOutMax=[]  bOutMin=[]  bOutMax=[]  cOutMin=[]  cOutMax=[]  KbOutMin=[]  KbOutMax=[]  KtOutMin=[]  KtOutMax=[]  IntegratorOutMin=[]  IntegratorOutMax=[]  FilterOutMin=[]  FilterOutMax=[]  SumOutMin=[]  SumOutMax=[]  Sum1OutMin=[]  Sum1OutMax=[]  Sum2OutMin=[]  Sum2OutMax=[]  Sum3OutMin=[]  Sum3OutMax=[]  SumI1OutMin=[]  SumI1OutMax=[]  SumI2OutMin=[]  SumI2OutMax=[]  SumI3OutMin=[]  SumI3OutMax=[]  SumDOutMin=[]  SumDOutMax=[]  SaturationOutMin=[]  SaturationOutMax=[]  IntegratorContinuousStateAttributes=''  IntegratorStateMustResolveToSignalObject=off  IntegratorRTWStateStorageClass=Auto  FilterContinuousStateAttributes=''  FilterStateMustResolveToSignalObject=off  FilterRTWStateStorageClass=Auto  DifferentiatorICPrevScaledInput=0  DifferentiatorOutMin=[]  DifferentiatorOutMax=[]  FilterDiffOutCoefMin=[]  FilterDiffOutCoefMax=[]  SumDenOutMin=[]  SumDenOutMax=[]  SumNumOutMin=[]  SumNumOutMax=[]  ReciprocalOutMin=[]  ReciprocalOutMax=[]  DivideOutMin=[]  DivideOutMax=[]  TunerSelectOption=Transfer Function Based (PID Tuner App)
  cfblk8 : simulink/Discrete/Transfer Fcn Real Zero  ZeroZ=0.75  ICPrevInput=0.0  DoSatur=off
      settings: SourceProductName=Simulink  SourceProductBaseCode=SL
  cfblk9 : simulink/Discrete/Transfer Fcn Real Zero  ZeroZ=0.75  ICPrevInput=0.0  DoSatur=off
      settings: SourceProductName=Simulink  SourceProductBaseCode=SL
  cfblk2 : Outport
  cfblk15 : Outport  Port=2
  wires:
  cfblk17/1(cfblk2) -> cfblk10/1
  cfblk17/2(cfblk12) -> cfblk9/1
  cfblk13/1 -> cfblk5/1
  cfblk4/1 -> cfblk8/1
  cfblk6/1 -> cfblk3/1
  cfblk1/1 -> cfblk11/1
  cfblk16/1(cfblk2) -> cfblk6/1
  cfblk10/1 -> cfblk15/1
  cfblk5/1 -> cfblk16/1(cfblk1)
  cfblk14/1 -> cfblk4/1
  cfblk12/1 -> cfblk16/2(cfblk11)
  cfblk9/1 -> cfblk2/1
  cfblk3/1 -> cfblk7/1
  cfblk16/2(cfblk12) -> cfblk4/2, cfblk7/2
  cfblk11/1 -> cfblk16/Action
  cfblk11/2 -> cfblk17/Action
  cfblk8/1 -> cfblk18/1
  cfblk18/1 -> cfblk17/1(cfblk1)

== system sampleModel2431_slicer/cfblk251 ==
  cfblk1 : Inport
  cfblk8 : Inport  Port=2
  Action Port : ActionPort  ActionType=then
  cfblk11 : Subsystem  TreatAsAtomicUnit=on
  cfblk12 : Subsystem  TreatAsAtomicUnit=on
  cfblk13 : Delay
  cfblk14 : Delay
  cfblk3 : Delay
  cfblk4 : DiscreteFir
  cfblk5 : simulink/Discrete/Transfer Fcn First Order  PoleZ=0.95  ICPrevOutput=0.0  DoSatur=off
      settings: SourceProductName=Simulink
  cfblk6 : simulink/Continuous/PID Controller (2DOF)  Controller=PID  TimeDomain=Discrete-time  SampleTime=-1  IntegratorMethod=Forward Euler  FilterMethod=Forward Euler  Form=Parallel  UseFilter=on  ControllerParametersSource=internal  P=1  I=1  D=0  N=100  b=1  c=1  InitialConditionSource=internal  InitialConditionForIntegrator=0  InitialConditionForFilter=0  ExternalReset=none  LimitOutput=off  UpperSaturationLimit=inf  LowerSaturationLimit=-inf  LinearizeAsGain=off  AntiWindupMode=none  Kb=1  TrackingMode=off  Kt=1  PParamMin=[]  PParamMax=[]  IParamMin=[]  IParamMax=[]  DParamMin=[]  DParamMax=[]  NParamMin=[]  NParamMax=[]  bParamMin=[]  bParamMax=[]  cParamMin=[]  cParamMax=[]  KbParamMin=[]  KbParamMax=[]  KtParamMin=[]  KtParamMax=[]  POutMin=[]  POutMax=[]  IOutMin=[]  IOutMax=[]  DOutMin=[]  DOutMax=[]  NOutMin=[]  NOutMax=[]  bOutMin=[]  bOutMax=[]  cOutMin=[]  cOutMax=[]  KbOutMin=[]  KbOutMax=[]  KtOutMin=[]  KtOutMax=[]  IntegratorOutMin=[]  IntegratorOutMax=[]  FilterOutMin=[]  FilterOutMax=[]  SumOutMin=[]  SumOutMax=[]  Sum1OutMin=[]  Sum1OutMax=[]  Sum2OutMin=[]  Sum2OutMax=[]  Sum3OutMin=[]  Sum3OutMax=[]  SumI1OutMin=[]  SumI1OutMax=[]  SumI2OutMin=[]  SumI2OutMax=[]  SumI3OutMin=[]  SumI3OutMax=[]  SumDOutMin=[]  SumDOutMax=[]  SaturationOutMin=[]  SaturationOutMax=[]  IntegratorContinuousStateAttributes=''  IntegratorStateMustResolveToSignalObject=off  IntegratorRTWStateStorageClass=Auto  FilterContinuousStateAttributes=''  FilterStateMustResolveToSignalObject=off  FilterRTWStateStorageClass=Auto  DifferentiatorICPrevScaledInput=0  DifferentiatorOutMin=[]  DifferentiatorOutMax=[]  FilterDiffOutCoefMin=[]  FilterDiffOutCoefMax=[]  SumDenOutMin=[]  SumDenOutMax=[]  SumNumOutMin=[]  SumNumOutMax=[]  ReciprocalOutMin=[]  ReciprocalOutMax=[]  DivideOutMin=[]  DivideOutMax=[]  TunerSelectOption=Transfer Function Based (PID Tuner App)
  cfblk7 : If  SampleTime=1
  cfblk2 : Outport
  cfblk9 : Outport  Port=2
  cfblk10 : Outport  Port=3
  wires:
  cfblk1/1 -> cfblk3/1
  cfblk4/1 -> cfblk6/1
  cfblk11/1(cfblk2) -> cfblk9/1
  cfblk6/1 -> cfblk10/1, cfblk5/1, cfblk14/1
  cfblk3/1 -> cfblk12/1(cfblk1)
  cfblk12/2(cfblk9) -> cfblk11/1(cfblk1)
  cfblk5/1 -> cfblk11/2(cfblk11)
  cfblk12/3(cfblk10) -> cfblk2/1
  cfblk8/1 -> cfblk6/2, cfblk12/2(cfblk8)
  cfblk7/1 -> cfblk11/Action
  cfblk7/2 -> cfblk12/Action
  cfblk12/1(cfblk2) -> cfblk13/1
  cfblk13/1 -> cfblk7/1
  cfblk14/1 -> cfblk4/1

== system sampleModel2431_slicer/cfblk252 ==
  cfblk1 : Inport
  cfblk10 : Inport  Port=2
  Action Port : ActionPort  ActionType=else
  cfblk11 : Delay
  cfblk12 : Delay
  cfblk3 : UnitDelay  SampleTime=-1
  cfblk4 : DiscreteStateSpace  SampleTime=-1
  cfblk5 : DiscreteIntegrator  SampleTime=-1  ICPrevOutput=DiscIntNeverNeededParam  ICPrevScaledInput=DiscIntNeverNeededParam
  cfblk6 : simulink/Continuous/PID Controller  Controller=PID  TimeDomain=Discrete-time  SampleTime=-1  IntegratorMethod=Forward Euler  FilterMethod=Forward Euler  Form=Parallel  UseFilter=on  ControllerParametersSource=internal  P=1  I=1  D=0  N=100  InitialConditionSource=internal  InitialConditionForIntegrator=0  InitialConditionForFilter=0  ExternalReset=none  LimitOutput=off  UpperSaturationLimit=inf  LowerSaturationLimit=-inf  LinearizeAsGain=off  AntiWindupMode=none  Kb=1  TrackingMode=off  Kt=1  PParamMin=[]  PParamMax=[]  IParamMin=[]  IParamMax=[]  DParamMin=[]  DParamMax=[]  NParamMin=[]  NParamMax=[]  KbParamMin=[]  KbParamMax=[]  KtParamMin=[]  KtParamMax=[]  POutMin=[]  POutMax=[]  IOutMin=[]  IOutMax=[]  DOutMin=[]  DOutMax=[]  NOutMin=[]  NOutMax=[]  KbOutMin=[]  KbOutMax=[]  KtOutMin=[]  KtOutMax=[]  IntegratorOutMin=[]  IntegratorOutMax=[]  FilterOutMin=[]  FilterOutMax=[]  SumOutMin=[]  SumOutMax=[]  SumI1OutMin=[]  SumI1OutMax=[]  SumI2OutMin=[]  SumI2OutMax=[]  SumI3OutMin=[]  SumI3OutMax=[]  SumDOutMin=[]  SumDOutMax=[]  SaturationOutMin=[]  SaturationOutMax=[]  IntegratorContinuousStateAttributes=''  IntegratorStateMustResolveToSignalObject=off  IntegratorRTWStateStorageClass=Auto  FilterContinuousStateAttributes=''  FilterStateMustResolveToSignalObject=off  FilterRTWStateStorageClass=Auto  DifferentiatorICPrevScaledInput=0  DifferentiatorOutMin=[]  DifferentiatorOutMax=[]  FilterDiffOutCoefMin=[]  FilterDiffOutCoefMax=[]  SumDenOutMin=[]  SumDenOutMax=[]  SumNumOutMin=[]  SumNumOutMax=[]  ReciprocalOutMin=[]  ReciprocalOutMax=[]  DivideOutMin=[]  DivideOutMax=[]  TunerSelectOption=Transfer Function Based (PID Tuner App)
  cfblk7 : simulink/Continuous/PID Controller  Controller=PID  TimeDomain=Discrete-time  SampleTime=-1  IntegratorMethod=Forward Euler  FilterMethod=Forward Euler  Form=Parallel  UseFilter=on  ControllerParametersSource=internal  P=1  I=1  D=0  N=100  InitialConditionSource=internal  InitialConditionForIntegrator=0  InitialConditionForFilter=0  ExternalReset=none  LimitOutput=off  UpperSaturationLimit=inf  LowerSaturationLimit=-inf  LinearizeAsGain=off  AntiWindupMode=none  Kb=1  TrackingMode=off  Kt=1  PParamMin=[]  PParamMax=[]  IParamMin=[]  IParamMax=[]  DParamMin=[]  DParamMax=[]  NParamMin=[]  NParamMax=[]  KbParamMin=[]  KbParamMax=[]  KtParamMin=[]  KtParamMax=[]  POutMin=[]  POutMax=[]  IOutMin=[]  IOutMax=[]  DOutMin=[]  DOutMax=[]  NOutMin=[]  NOutMax=[]  KbOutMin=[]  KbOutMax=[]  KtOutMin=[]  KtOutMax=[]  IntegratorOutMin=[]  IntegratorOutMax=[]  FilterOutMin=[]  FilterOutMax=[]  SumOutMin=[]  SumOutMax=[]  SumI1OutMin=[]  SumI1OutMax=[]  SumI2OutMin=[]  SumI2OutMax=[]  SumI3OutMin=[]  SumI3OutMax=[]  SumDOutMin=[]  SumDOutMax=[]  SaturationOutMin=[]  SaturationOutMax=[]  IntegratorContinuousStateAttributes=''  IntegratorStateMustResolveToSignalObject=off  IntegratorRTWStateStorageClass=Auto  FilterContinuousStateAttributes=''  FilterStateMustResolveToSignalObject=off  FilterRTWStateStorageClass=Auto  DifferentiatorICPrevScaledInput=0  DifferentiatorOutMin=[]  DifferentiatorOutMax=[]  FilterDiffOutCoefMin=[]  FilterDiffOutCoefMax=[]  SumDenOutMin=[]  SumDenOutMax=[]  SumNumOutMin=[]  SumNumOutMax=[]  ReciprocalOutMin=[]  ReciprocalOutMax=[]  DivideOutMin=[]  DivideOutMax=[]  TunerSelectOption=Transfer Function Based (PID Tuner App)
  cfblk8 : simulink/Continuous/PID Controller (2DOF)  Controller=PID  TimeDomain=Discrete-time  SampleTime=-1  IntegratorMethod=Forward Euler  FilterMethod=Forward Euler  Form=Parallel  UseFilter=on  ControllerParametersSource=internal  P=1  I=1  D=0  N=100  b=1  c=1  InitialConditionSource=internal  InitialConditionForIntegrator=0  InitialConditionForFilter=0  ExternalReset=none  LimitOutput=off  UpperSaturationLimit=inf  LowerSaturationLimit=-inf  LinearizeAsGain=off  AntiWindupMode=none  Kb=1  TrackingMode=off  Kt=1  PParamMin=[]  PParamMax=[]  IParamMin=[]  IParamMax=[]  DParamMin=[]  DParamMax=[]  NParamMin=[]  NParamMax=[]  bParamMin=[]  bParamMax=[]  cParamMin=[]  cParamMax=[]  KbParamMin=[]  KbParamMax=[]  KtParamMin=[]  KtParamMax=[]  POutMin=[]  POutMax=[]  IOutMin=[]  IOutMax=[]  DOutMin=[]  DOutMax=[]  NOutMin=[]  NOutMax=[]  bOutMin=[]  bOutMax=[]  cOutMin=[]  cOutMax=[]  KbOutMin=[]  KbOutMax=[]  KtOutMin=[]  KtOutMax=[]  IntegratorOutMin=[]  IntegratorOutMax=[]  FilterOutMin=[]  FilterOutMax=[]  SumOutMin=[]  SumOutMax=[]  Sum1OutMin=[]  Sum1OutMax=[]  Sum2OutMin=[]  Sum2OutMax=[]  Sum3OutMin=[]  Sum3OutMax=[]  SumI1OutMin=[]  SumI1OutMax=[]  SumI2OutMin=[]  SumI2OutMax=[]  SumI3OutMin=[]  SumI3OutMax=[]  SumDOutMin=[]  SumDOutMax=[]  SaturationOutMin=[]  SaturationOutMax=[]  IntegratorContinuousStateAttributes=''  IntegratorStateMustResolveToSignalObject=off  IntegratorRTWStateStorageClass=Auto  FilterContinuousStateAttributes=''  FilterStateMustResolveToSignalObject=off  FilterRTWStateStorageClass=Auto  DifferentiatorICPrevScaledInput=0  DifferentiatorOutMin=[]  DifferentiatorOutMax=[]  FilterDiffOutCoefMin=[]  FilterDiffOutCoefMax=[]  SumDenOutMin=[]  SumDenOutMax=[]  SumNumOutMin=[]  SumNumOutMax=[]  ReciprocalOutMin=[]  ReciprocalOutMax=[]  DivideOutMin=[]  DivideOutMax=[]  TunerSelectOption=Transfer Function Based (PID Tuner App)
  cfblk9 : Delay
  cfblk2 : Outport
  wires:
  cfblk5/1 -> cfblk4/1
  cfblk7/1 -> cfblk2/1
  cfblk3/1 -> cfblk9/1
  cfblk4/1 -> cfblk7/1
  cfblk10/1 -> cfblk5/1
  cfblk1/1 -> cfblk8/2
  cfblk8/1 -> cfblk6/1
  cfblk6/1 -> cfblk11/1
  cfblk11/1 -> cfblk8/1
  cfblk9/1 -> cfblk12/1
  cfblk12/1 -> cfblk3/1

== system sampleModel2431_slicer/cfblk201/cfblk14 ==
  cfblk1 : Inport
  cfblk13 : Inport  Port=2
  Action Port : ActionPort  ActionType=then
  cfblk10 : DiscreteZeroPole  Poles=[0 0.5]  Gain=1  SampleTime=-1
  cfblk11 : DiscreteZeroPole  Poles=[0 0.5]  Gain=1  SampleTime=-1
  cfblk12 : simulink/Discrete/Difference  ICPrevInput=0.0  OutMin=[]  OutMax=[]  OutDataTypeStr=Inherit: Inherit via back propagation  OutDataType=fixdt(1, 16)  OutScaling=2^-10  DoSatur=off
  cfblk15 : Delay
  cfblk3 : DiscreteStateSpace  SampleTime=-1
  cfblk4 : simulink/Continuous/PID Controller (2DOF)  Controller=PID  TimeDomain=Discrete-time  SampleTime=-1  IntegratorMethod=Forward Euler  FilterMethod=Forward Euler  Form=Parallel  UseFilter=on  ControllerParametersSource=internal  P=1  I=1  D=0  N=100  b=1  c=1  InitialConditionSource=internal  InitialConditionForIntegrator=0  InitialConditionForFilter=0  ExternalReset=none  LimitOutput=off  UpperSaturationLimit=inf  LowerSaturationLimit=-inf  LinearizeAsGain=off  AntiWindupMode=none  Kb=1  TrackingMode=off  Kt=1  PParamMin=[]  PParamMax=[]  IParamMin=[]  IParamMax=[]  DParamMin=[]  DParamMax=[]  NParamMin=[]  NParamMax=[]  bParamMin=[]  bParamMax=[]  cParamMin=[]  cParamMax=[]  KbParamMin=[]  KbParamMax=[]  KtParamMin=[]  KtParamMax=[]  POutMin=[]  POutMax=[]  IOutMin=[]  IOutMax=[]  DOutMin=[]  DOutMax=[]  NOutMin=[]  NOutMax=[]  bOutMin=[]  bOutMax=[]  cOutMin=[]  cOutMax=[]  KbOutMin=[]  KbOutMax=[]  KtOutMin=[]  KtOutMax=[]  IntegratorOutMin=[]  IntegratorOutMax=[]  FilterOutMin=[]  FilterOutMax=[]  SumOutMin=[]  SumOutMax=[]  Sum1OutMin=[]  Sum1OutMax=[]  Sum2OutMin=[]  Sum2OutMax=[]  Sum3OutMin=[]  Sum3OutMax=[]  SumI1OutMin=[]  SumI1OutMax=[]  SumI2OutMin=[]  SumI2OutMax=[]  SumI3OutMin=[]  SumI3OutMax=[]  SumDOutMin=[]  SumDOutMax=[]  SaturationOutMin=[]  SaturationOutMax=[]  IntegratorContinuousStateAttributes=''  IntegratorStateMustResolveToSignalObject=off  IntegratorRTWStateStorageClass=Auto  FilterContinuousStateAttributes=''  FilterStateMustResolveToSignalObject=off  FilterRTWStateStorageClass=Auto  DifferentiatorICPrevScaledInput=0  DifferentiatorOutMin=[]  DifferentiatorOutMax=[]  FilterDiffOutCoefMin=[]  FilterDiffOutCoefMax=[]  SumDenOutMin=[]  SumDenOutMax=[]  SumNumOutMin=[]  SumNumOutMax=[]  ReciprocalOutMin=[]  ReciprocalOutMax=[]  DivideOutMin=[]  DivideOutMax=[]  TunerSelectOption=Transfer Function Based (PID Tuner App)
  cfblk5 : DiscreteZeroPole  Poles=[0 0.5]  Gain=1  SampleTime=-1
  cfblk6 : UnitDelay  SampleTime=-1
  cfblk7 : DiscreteIntegrator  SampleTime=-1  ICPrevOutput=DiscIntNeverNeededParam  ICPrevScaledInput=DiscIntNeverNeededParam
  cfblk8 : DiscreteFilter
  cfblk9 : DiscreteTransferFcn
  cfblk2 : Outport
  cfblk14 : Outport  Port=2
  wires:
  cfblk5/1 -> cfblk6/1
  cfblk4/1 -> cfblk7/1
  cfblk9/1 -> cfblk5/1
  cfblk13/1 -> cfblk12/1
  cfblk3/1 -> cfblk2/1
  cfblk1/1 -> cfblk10/1, cfblk4/2
  cfblk12/1 -> cfblk3/1
  cfblk10/1 -> cfblk9/1
  cfblk8/1 -> cfblk11/1
  cfblk7/1 -> cfblk14/1
  cfblk6/1 -> cfblk4/1
  cfblk11/1 -> cfblk15/1
  cfblk15/1 -> cfblk8/1

== system sampleModel2431_slicer/cfblk201/cfblk15 ==
  cfblk1 : Inport
  cfblk13 : Inport  Port=2
  cfblk14 : Inport  Port=3
  cfblk15 : Inport  Port=4
  cfblk16 : Inport  Port=5
  Action Port : ActionPort  ActionType=else
  cfblk10 : DiscreteTransferFcn
  cfblk11 : UnitDelay  SampleTime=-1
  cfblk12 : DiscreteZeroPole  Poles=[0 0.5]  Gain=1  SampleTime=-1
  cfblk18 : Delay
  cfblk3 : DiscreteStateSpace  SampleTime=-1
  cfblk4 : simulink/Discrete/Tapped Delay  vinit=0.0  samptime=-1  NumDelays=1  DelayOrder=Oldest  includeCurrent=off
  cfblk5 : UnitDelay  SampleTime=-1
  cfblk6 : simulink/Continuous/PID Controller  Controller=PID  TimeDomain=Discrete-time  SampleTime=-1  IntegratorMethod=Forward Euler  FilterMethod=Forward Euler  Form=Parallel  UseFilter=on  ControllerParametersSource=internal  P=1  I=1  D=0  N=100  InitialConditionSource=internal  InitialConditionForIntegrator=0  InitialConditionForFilter=0  ExternalReset=none  LimitOutput=off  UpperSaturationLimit=inf  LowerSaturationLimit=-inf  LinearizeAsGain=off  AntiWindupMode=none  Kb=1  TrackingMode=off  Kt=1  PParamMin=[]  PParamMax=[]  IParamMin=[]  IParamMax=[]  DParamMin=[]  DParamMax=[]  NParamMin=[]  NParamMax=[]  KbParamMin=[]  KbParamMax=[]  KtParamMin=[]  KtParamMax=[]  POutMin=[]  POutMax=[]  IOutMin=[]  IOutMax=[]  DOutMin=[]  DOutMax=[]  NOutMin=[]  NOutMax=[]  KbOutMin=[]  KbOutMax=[]  KtOutMin=[]  KtOutMax=[]  IntegratorOutMin=[]  IntegratorOutMax=[]  FilterOutMin=[]  FilterOutMax=[]  SumOutMin=[]  SumOutMax=[]  SumI1OutMin=[]  SumI1OutMax=[]  SumI2OutMin=[]  SumI2OutMax=[]  SumI3OutMin=[]  SumI3OutMax=[]  SumDOutMin=[]  SumDOutMax=[]  SaturationOutMin=[]  SaturationOutMax=[]  IntegratorContinuousStateAttributes=''  IntegratorStateMustResolveToSignalObject=off  IntegratorRTWStateStorageClass=Auto  FilterContinuousStateAttributes=''  FilterStateMustResolveToSignalObject=off  FilterRTWStateStorageClass=Auto  DifferentiatorICPrevScaledInput=0  DifferentiatorOutMin=[]  DifferentiatorOutMax=[]  FilterDiffOutCoefMin=[]  FilterDiffOutCoefMax=[]  SumDenOutMin=[]  SumDenOutMax=[]  SumNumOutMin=[]  SumNumOutMax=[]  ReciprocalOutMin=[]  ReciprocalOutMax=[]  DivideOutMin=[]  DivideOutMax=[]  TunerSelectOption=Transfer Function Based (PID Tuner App)
  cfblk7 : Delay  ShowEnablePort=on
      settings: InputPortMap=u0,e6
  cfblk8 : Delay  DelayLengthSource=Input port
      settings: InputPortMap=u0,p1
  cfblk9 : DiscreteFir
  cfblk2 : Outport
  cfblk17 : Outport  Port=2
  wires:
  cfblk15/1 -> cfblk7/1
  cfblk5/1 -> cfblk7/2
  cfblk6/1 -> cfblk3/1
  cfblk7/1 -> cfblk17/1
  cfblk9/1 -> cfblk11/1
  cfblk4/1 -> cfblk12/1
  cfblk12/1 -> cfblk10/1
  cfblk3/1 -> cfblk9/1
  cfblk13/1 -> cfblk8/1
  cfblk14/1 -> cfblk6/1
  cfblk1/1 -> cfblk2/1
  cfblk8/1 -> cfblk5/1
  cfblk11/1 -> cfblk8/2
  cfblk10/1 -> cfblk18/1
  cfblk18/1 -> cfblk4/1

== system sampleModel2431_slicer/cfblk201/cfblk16 ==
  cfblk1 : Inport
  Action Port : ActionPort  ActionType=then
  cfblk3 : Delay
  cfblk4 : Delay  ShowEnablePort=on
      settings: InputPortMap=u0,e6
  cfblk5 : DiscreteTransferFcn
  cfblk8 : Delay
  cfblk2 : Outport
  cfblk6 : Outport  Port=2
  cfblk7 : Outport  Port=3
  wires:
  cfblk1/1 -> cfblk4/2
  cfblk3/1 -> cfblk2/1, cfblk7/1
  cfblk4/1 -> cfblk6/1, cfblk5/1, cfblk3/1
  cfblk5/1 -> cfblk8/1
  cfblk8/1 -> cfblk4/1
